simulink subsystem "subsys_calcul_capteurs"  (R2021b)
settings: Solver=VariableStepAuto  StartTime=0.0  StopTime=10.0  RelTol=1e-3
settings Model: Creator=antho  LastModifiedBy=alexi

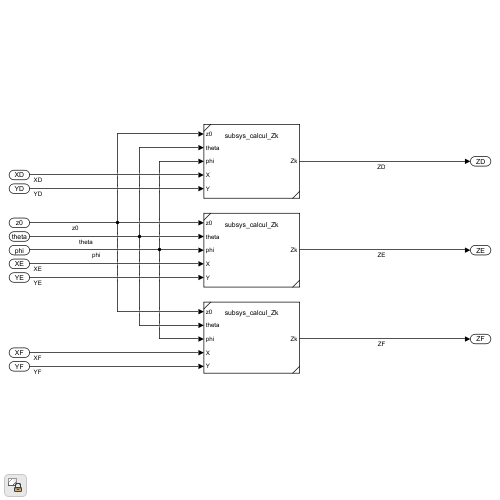
[thumbnail: Simulink's stored preview of the top-level diagram]
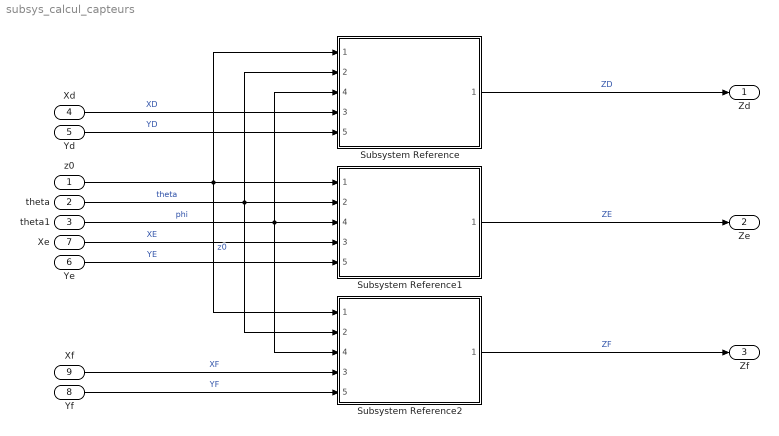
== system subsys_calcul_capteurs ==
  z0 : Inport
  theta : Inport  Port=2
  theta1 : Inport  Port=3
  Xd : Inport  Port=4
  Yd : Inport  Port=5
  Ye : Inport  Port=6
  Xe : Inport  Port=7
  Yf : Inport  Port=8
  Xf : Inport  Port=9
  Subsystem Reference : Subsystem  ReferencedSubsystem=subsys_calcul_Zk
      settings: PortSchema="{\"entries\":[{\"content\":{\"sides\":[{\"content\":{\"connectorIds\":[\"In1\",\"In2\",\"In4\",\"In3\",\"In5\"]},\"type\":\"ConnectorPlacement.EquallySpacedRectSide\",\"uuid\":\"58a7cade-cf80-43c0-946c-336fdbd8c2a7\"},{\"content\":{\"connectorIds\":[\"Out1\"],\"side\":\"RIGHT\"},\"type\":\"ConnectorPlacement.EquallySpacedRectSide\",\"uuid\":\"9a223902-f7c0-4b06-b74a-0bbf211990a4\"},{\"content\":{\"connectorIds\":[],\"side\":\"TOP\"},\"type\":\"ConnectorPlacement.EquallySpacedRectSide\",\"uuid\":\"8d5abb67-7ecf-4602-9715-44c58f718e55\"}]},\"type\":\"ConnectorPlacement.EquallySpacedConnector\",\"uuid\":\"bbfaaa32-0739-40af-9581-6fc28608cdbf\"}],\"packageUris\":[\"http://schema.mathworks.com/mf0/Connector/R2020b\"],\"version\":\"1.0\"}"
  Subsystem Reference1 : Subsystem  ReferencedSubsystem=subsys_calcul_Zk
      settings: PortSchema="{\"entries\":[{\"content\":{\"sides\":[{\"content\":{\"connectorIds\":[\"In1\",\"In2\",\"In4\",\"In3\",\"In5\"]},\"type\":\"ConnectorPlacement.EquallySpacedRectSide\",\"uuid\":\"58a7cade-cf80-43c0-946c-336fdbd8c2a7\"},{\"content\":{\"connectorIds\":[\"Out1\"],\"side\":\"RIGHT\"},\"type\":\"ConnectorPlacement.EquallySpacedRectSide\",\"uuid\":\"9a223902-f7c0-4b06-b74a-0bbf211990a4\"},{\"content\":{\"connectorIds\":[],\"side\":\"TOP\"},\"type\":\"ConnectorPlacement.EquallySpacedRectSide\",\"uuid\":\"8d5abb67-7ecf-4602-9715-44c58f718e55\"}]},\"type\":\"ConnectorPlacement.EquallySpacedConnector\",\"uuid\":\"bbfaaa32-0739-40af-9581-6fc28608cdbf\"}],\"packageUris\":[\"http://schema.mathworks.com/mf0/Connector/R2020b\"],\"version\":\"1.0\"}"
  Subsystem Reference2 : Subsystem  ReferencedSubsystem=subsys_calcul_Zk
      settings: PortSchema="{\"entries\":[{\"content\":{\"sides\":[{\"content\":{\"connectorIds\":[\"In1\",\"In2\",\"In4\",\"In3\",\"In5\"]},\"type\":\"ConnectorPlacement.EquallySpacedRectSide\",\"uuid\":\"58a7cade-cf80-43c0-946c-336fdbd8c2a7\"},{\"content\":{\"connectorIds\":[\"Out1\"],\"side\":\"RIGHT\"},\"type\":\"ConnectorPlacement.EquallySpacedRectSide\",\"uuid\":\"9a223902-f7c0-4b06-b74a-0bbf211990a4\"},{\"content\":{\"connectorIds\":[],\"side\":\"TOP\"},\"type\":\"ConnectorPlacement.EquallySpacedRectSide\",\"uuid\":\"8d5abb67-7ecf-4602-9715-44c58f718e55\"}]},\"type\":\"ConnectorPlacement.EquallySpacedConnector\",\"uuid\":\"bbfaaa32-0739-40af-9581-6fc28608cdbf\"}],\"packageUris\":[\"http://schema.mathworks.com/mf0/Connector/R2020b\"],\"version\":\"1.0\"}"
  Zd : Outport
  Ze : Outport  Port=2
  Zf : Outport  Port=3
  wires:
  z0/1 -> Subsystem Reference1/1, Subsystem Reference/1, Subsystem Reference2/1  "z0"
  theta/1 -> Subsystem Reference1/2, Subsystem Reference/2, Subsystem Reference2/2  "theta"
  theta1/1 -> Subsystem Reference2/4, Subsystem Reference1/4, Subsystem Reference/4  "phi"
  Xd/1 -> Subsystem Reference/3  "XD"
  Xe/1 -> Subsystem Reference1/3  "XE"
  Yd/1 -> Subsystem Reference/5  "YD"
  Ye/1 -> Subsystem Reference1/5  "YE"
  Xf/1 -> Subsystem Reference2/3  "XF"
  Yf/1 -> Subsystem Reference2/5  "YF"
  Subsystem Reference/1 -> Zd/1  "ZD"
  Subsystem Reference2/1 -> Zf/1  "ZF"
  Subsystem Reference1/1 -> Ze/1  "ZE"
